simulink model "Demo3"  (Simulink 6.5)
settings: Solver=ode23t  SolverMode=SingleTasking  StartTime=0.0  StopTime=.1  RelTol=1e-3
undefined symbols (not defined in the file): powergui
libraries: powerlib x17, powerlib_extras x1
settings Model: Creator=sybille  LastModifiedBy=PC_0  ExtModeTrigMode=oneshot  ExtModeArmWhenConnect=off  ExtModeAutoUpdateStatusClock=off
settings SolverCC: MaxOrder=1
settings DataIOCC: LimitDataPoints=off  SaveOutput=off  SaveTime=off  SignalLoggingName=sigsOut
settings OptimizationCC: BlockReduction=off  BooleanDataType=off  InlineInvariantSignals=on
settings DebuggingCC: CheckExecutionContextPreStartOutputMsg=on  CheckExecutionContextRuntimeOutputMsg=on  SolverPrmCheckMsg=none  MultiTaskDSMMsg=warning  MultiTaskCondExecSysMsg=none  SigSpecEnsureSampleTimeMsg=none  UnconnectedInputMsg=none  UnconnectedOutputMsg=none  StrictBusMsg=None
settings HardwareCC: TargetUnknown=on
settings RTWCC: IncludeERTFirstTime=on

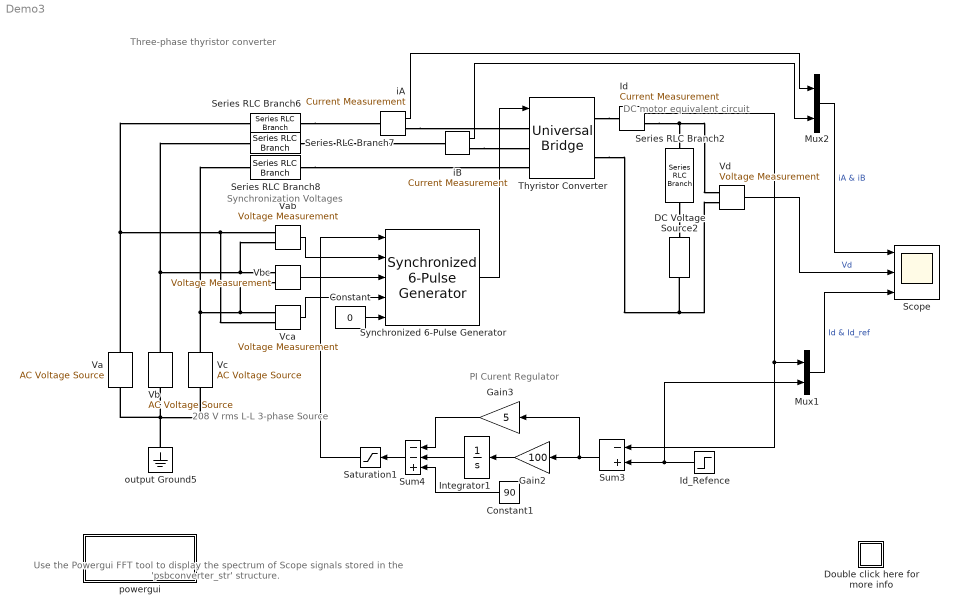
== system Demo3 ==
  note: Synchronization Voltages
  note: DC motor equivalent circuit
  note: PI Curent Regulator
  note: Three-phase thyristor converter
  note: 208 V rms L-L
      | 3-phase Source
  note: Use the Powergui FFT tool to display
      | the spectrum of Scope  signals stored in
      | the 'psbconverter_str' structure.
  Constant : Constant  Value=0  OutDataType=sfix(16)  ConRadixGroup=Use specified scaling  OutScaling=2^0  SampleTime=inf  FramePeriod=inf
  Constant1 : Constant  Orientation=left  Value=90  OutDataType=sfix(16)  ConRadixGroup=Use specified scaling  OutScaling=2^0  SampleTime=inf  FramePeriod=inf
  DC Voltage Source2 : powerlib/Electrical Sources/DC Voltage Source  Description=source block  Orientation=up  DialogController=PMDialogs.PMDefaultMaskDlg  SystemSampleTime=-1  Amplitude=120  Measurements=None
      settings: AttributesFormatString=\n
  Double click here for more info : Subsystem
      settings: OpenFcn=showdemo(bdroot(gcb))
      mask Display: disp('?')
  Gain2 : Gain  Orientation=left  Gain=100  SaturateOnIntegerOverflow=on
  Gain3 : Gain  Orientation=left  Gain=5  SaturateOnIntegerOverflow=on
  Id : powerlib/Measurements/Current Measurement  Tag=PoWeRsYsTeMmEaSuReMeNt  DialogController=PMDialogs.PMDefaultMaskDlg  SystemSampleTime=-1  PhasorSimulation=off  OutputType=Complex  PSBequivalent=0
  Id_Refence : Step  Orientation=left  Time=0.04  Before=10  After=25  SampleTime=0
  Integrator1 : Integrator  Orientation=left  InitialCondition=20  LimitOutput=on  UpperSaturationLimit=160  LowerSaturationLimit=20
  Mux1 : Mux  Inputs=2
  Mux2 : Mux  Inputs=2
  Saturation1 : Saturate  Orientation=left  UpperLimit=160  LowerLimit=20
  Scope : Scope  NumInputPorts=3
      settings: TimeRange=0.1  YMin=-50~-200~-3.20216e-017  YMax=50~400~40  SaveName=psbconverter_str  SampleInput=on  SampleTime=1/60/512
  Series RLC Branch2 : powerlib/Elements/Series RLC Branch  Orientation=down  DialogController=PMDialogs.PMDefaultMaskDlg  PhysicalDomain=powersysdomain  SubClassName=unknown  LeftPortType=p1  RightPortType=p1  LConnTagsString=__new0  RConnTagsString=__new0  BranchType=RL  Resistance=1  Inductance=20e-3  SetiL0=off  InitialCurrent=0  Capacitance=[]  Setx0=off  InitialVoltage=0  Measurements=None
  Series RLC Branch6 : powerlib/Elements/Series RLC Branch  DialogController=PMDialogs.PMDefaultMaskDlg  PhysicalDomain=powersysdomain  SubClassName=unknown  LeftPortType=p1  RightPortType=p1  LConnTagsString=__new0  RConnTagsString=__new0  BranchType=RL  Resistance=0.01  Inductance=1e-3  SetiL0=off  InitialCurrent=0  Capacitance=[]  Setx0=off  InitialVoltage=0  Measurements=None
  Series RLC Branch7 : powerlib/Elements/Series RLC Branch  DialogController=PMDialogs.PMDefaultMaskDlg  PhysicalDomain=powersysdomain  SubClassName=unknown  LeftPortType=p1  RightPortType=p1  LConnTagsString=__new0  RConnTagsString=__new0  BranchType=RL  Resistance=0.01  Inductance=1e-3  SetiL0=off  InitialCurrent=0  Capacitance=[]  Setx0=off  InitialVoltage=0  Measurements=None
  Series RLC Branch8 : powerlib/Elements/Series RLC Branch  DialogController=PMDialogs.PMDefaultMaskDlg  PhysicalDomain=powersysdomain  SubClassName=unknown  LeftPortType=p1  RightPortType=p1  LConnTagsString=__new0  RConnTagsString=__new0  BranchType=RL  Resistance=0.01  Inductance=1e-3  SetiL0=off  InitialCurrent=0  Capacitance=[]  Setx0=off  InitialVoltage=0  Measurements=None
  Sum3 : Sum  Orientation=left  Inputs=-+  SaturateOnIntegerOverflow=on  InputSameDT=on
  Sum4 : Sum  Orientation=left  Inputs=--+  SaturateOnIntegerOverflow=on  InputSameDT=on
  Synchronized 6-Pulse Generator : powerlib_extras/Control  Blocks/Synchronized 6-Pulse Generator  DialogController=PMDialogs.PMDefaultMaskDlg  SystemSampleTime=-1  freq=60  pwidth=10  Double_Pulse=on
  Thyristor Converter : powerlib/Power Electronics/Universal Bridge  DialogController=PMDialogs.PMDefaultMaskDlg  SystemSampleTime=-1  Arms=3  SnubberResistance=500  SnubberCapacitance=.1e-6  Device=Thyristors  Ron=1e-3  Lon=0  ForwardVoltages="[  0.8  0.8  ]"  ForwardVoltage=.8  GTOparameters=[ 10e-6 , 20e-6 ]  IGBTparameters=[ 1e-6 , 2e-6 ]  Measurements=None  converterType=Rectifier
  Va : powerlib/Electrical Sources/AC Voltage Source  Description=source block  Orientation=up  DialogController=PMDialogs.PMDefaultMaskDlg  SystemSampleTime=-1  Amplitude=208*sqrt(2/3)  Phase=0  Frequency=60  SampleTime=0  Measurements=None
      settings: AttributesFormatString=\n
  Vab : powerlib/Measurements/Voltage Measurement  Tag=PoWeRsYsTeMmEaSuReMeNt  DialogController=PMDialogs.PMDefaultMaskDlg  SystemSampleTime=-1  PhasorSimulation=off  OutputType=Complex  PSBequivalent=0
  Vb : powerlib/Electrical Sources/AC Voltage Source  Description=source block  Orientation=up  DialogController=PMDialogs.PMDefaultMaskDlg  SystemSampleTime=-1  Amplitude=208*sqrt(2/3)  Phase=-120  Frequency=60  SampleTime=0  Measurements=None
      settings: AttributesFormatString=\n
  Vbc : powerlib/Measurements/Voltage Measurement  Tag=PoWeRsYsTeMmEaSuReMeNt  DialogController=PMDialogs.PMDefaultMaskDlg  SystemSampleTime=-1  PhasorSimulation=off  OutputType=Complex  PSBequivalent=0
  Vc : powerlib/Electrical Sources/AC Voltage Source  Description=source block  Orientation=up  DialogController=PMDialogs.PMDefaultMaskDlg  SystemSampleTime=-1  Amplitude=208*sqrt(2/3)  Phase=120  Frequency=60  SampleTime=0  Measurements=None
      settings: AttributesFormatString=\n
  Vca : powerlib/Measurements/Voltage Measurement  Tag=PoWeRsYsTeMmEaSuReMeNt  DialogController=PMDialogs.PMDefaultMaskDlg  SystemSampleTime=-1  PhasorSimulation=off  OutputType=Complex  PSBequivalent=0
  Vd : powerlib/Measurements/Voltage Measurement  Tag=PoWeRsYsTeMmEaSuReMeNt  DialogController=PMDialogs.PMDefaultMaskDlg  SystemSampleTime=-1  PhasorSimulation=off  OutputType=Complex  PSBequivalent=0
  iA : powerlib/Measurements/Current Measurement  Tag=PoWeRsYsTeMmEaSuReMeNt  DialogController=PMDialogs.PMDefaultMaskDlg  SystemSampleTime=-1  PhasorSimulation=off  OutputType=Complex  PSBequivalent=0
  iB : powerlib/Measurements/Current Measurement  Tag=PoWeRsYsTeMmEaSuReMeNt  DialogController=PMDialogs.PMDefaultMaskDlg  SystemSampleTime=-1  PhasorSimulation=off  OutputType=Complex  PSBequivalent=0
  output Ground5 : powerlib/Elements/Ground  Orientation=down  DialogController=PMDialogs.PMDefaultMaskDlg  PhysicalDomain=powersysdomain  SubClassName=unknown  LeftPortType=p1  RightPortType=p1  LConnTagsString=a
  powergui : Subsystem  Priority=2  AncestorBlock=powerlib/powergui  InitFcn=powergui( 'InitFcn_Callback' , gcb , 0 , [ ] );  mask(PSB option menu block){SimulationMode=Continuous, SampleTime=0, echomessages=off, RestoreLinks=warning, x0status=blocks, Frange=[0:2:500], Ylog=off, Xlog=on, ShowGrid=off, save=off, variable=ZData, structure=psbconverter_str, ZoomFFT=on, StartTime=0.1-2/60, cycles=2, DisplayStyle=off, fundamental=60, FreqAxis=on, MaxFrequency=2000, frequencyindice=60, frequencyindicesteady=1, RmsSteady=1, display=off, Ts=0, frequency=60, methode=off, HookPort=off, Interpol=off}
      mask prompts: SimulationMode "Simulation mode"; SampleTime "Sample time Ts (when simulation mode is Discrete) (s)"; echomessages "Echo  Messages"; RestoreLinks "Restore disabled links"; x0status "Initial electrical states status"; Frange "Impedance tool: Frequency Range"; Ylog "Impedance tool: Log impedance"; Xlog "Impedance tool: log Frequency"; ShowGrid "Impedance tool: grid"; save "Impedance tool: Save Data To Workspace"; variable "Impedance tool: Variable Name"; structure "Structure Name (PSBFFTSCOPE)"; ZoomFFT "ZoomFFT (PSBFFTSCOPE)"; StartTime "Start Time (PSBFFTSCOPE)"; cycles "Cycles (PSBFFTSCOPE)"; DisplayStyle "Display style (PSBFFTSCOPE)"; fundamental "Fundamental (PSBFFTSCOPE)"; FreqAxis "Frequency Axis (PSBFFTSCOPE)"; MaxFrequency "Max Frequency (PSBFFTSCOPE)"; frequencyindice "Load flow frequency (Hz)"; frequencyindicesteady "Frequency indice (STEADYSTATE)"; RmsSteady "RMS display (STEADYSTATE)"; display "Display Results"; Ts "OBSOLETE 1"; frequency "Phasor frequency (Hz)"; methode "Phasor simulation"; HookPort "Hook port"; Interpol "Interpolate"
      mask init:
      | powerlibroot = which('powersysdomain');
      | PSBroot = powerlibroot(1:end-16);
      | %
      | switch SimulationMode
      | 	case 1
      | 		message=sprintf('Continuous');
      | 	case 2
      |         SampleTimeeval=evalin('base',SampleTime,'NaN');
      |         if isnan(SampleTimeeval)
      |             message=sprintf('Warning !!,\nUndefined sample time');
      |         else
      |             message=sprintf('Discrete,\nTs = %.4g s.',SampleTimeeval);
      |         end
      | 	case 3
      | 		message=sprintf('Phasors');
      | end
      | if strcmp(bdroot,'powerlib')
      |   message='powergui';
      | end
      | power_initmask();
      settings: CopyFcn=powergui( 'Copy_Callback' , gcb , 0 , [ ] );  ModelCloseFcn=powergui( 'CloseButton_Callback' , gcb , [ ] , [ ] );  PreSaveFcn=powergui( 'CloseButton_Callback' , gcb , [ ] , [ ] );  NameChangeFcn=powergui( 'NameChangeFcn_Callback' , gcb , 0 , [ ] );
      settings: DeleteFcn=|
      | powergui( 'Copy_Callback' , gcb , 1 , [ ] );
      | powergui( 'CloseButton_Callback' , gcb , [ ] , [ ] );
      settings: OpenFcn=|
      | if (power_openblockproxy ('secondary'))
      | powergui(gcb,'PM')
      | end;
      mask Help: web(psbhelp)
      mask StyleString: popup(Continuous|Discrete|Phasor),edit,checkbox,popup(yes|warning|no),popup(blocks|steady|zero),edit,checkbox,checkbox,checkbox,checkbox,edit,edit,checkbox,edit,edit,edit,edit,checkbox,edit,edit,edit,edit,checkbox,edit,edit,checkbox,checkbox,checkbox
      mask CallbackString: ||||||||||||||||||||||||||powergui('HookPort',[],[],gcb);|
      mask Display: disp(message)
  wires:
  Gain3/1 -> Sum4/1
  Constant1/1 -> Sum4/3
  Gain2/1 -> Integrator1/1
  Sum3/1 -> Gain3/1, Gain2/1
  Sum4/1 -> Saturation1/1
  Integrator1/1 -> Sum4/2
  Saturation1/1 -> Synchronized 6-Pulse Generator/1
  Id_Refence/1 -> Sum3/2, Mux1/2
  Mux2/1 -> Scope/1  "iA & iB"
  Mux1/1 -> Scope/3  "Id & Id_ref"
  Constant/1 -> Synchronized 6-Pulse Generator/5
  Id/1 -> Mux1/1, Sum3/1
  Vca/1 -> Synchronized 6-Pulse Generator/4
  Vbc/1 -> Synchronized 6-Pulse Generator/3
  Vab/1 -> Synchronized 6-Pulse Generator/2
  iA/1 -> Mux2/1
  iB/1 -> Mux2/2
  Vd/1 -> Scope/2  "Vd"
  Synchronized 6-Pulse Generator/1 -> Thyristor Converter/1
  connections:
  Thyristor Converter/RConn1 -- Id/LConn1
  output Ground5/LConn1 -- Vb/LConn1 -- Va/LConn1 -- Vc/LConn1
  Id/RConn1 -- Series RLC Branch2/LConn1 -- Vd/LConn1
  Series RLC Branch2/RConn1 -- DC Voltage Source2/RConn1
  Vb/RConn1 -- Vbc/LConn1 -- Vab/LConn2 -- Series RLC Branch7/LConn1
  Vc/RConn1 -- Vca/LConn1 -- Vbc/LConn2 -- Series RLC Branch8/LConn1
  Va/RConn1 -- Vab/LConn1 -- Vca/LConn2 -- Series RLC Branch6/LConn1
  Series RLC Branch8/RConn1 -- Thyristor Converter/LConn3
  Series RLC Branch6/RConn1 -- iA/LConn1
  iA/RConn1 -- Thyristor Converter/LConn1
  Series RLC Branch7/RConn1 -- iB/LConn1
  iB/RConn1 -- Thyristor Converter/LConn2
  Thyristor Converter/RConn2 -- DC Voltage Source2/LConn1 -- Vd/LConn2

== system Demo3/Double click here for more info ==
  note: This demonstration illustrates use of the Universal Bridge block to simulate a three-phase six-pulse
      | converter and harmonic analysis using the Powergui/FFT tool.
  note: Circuit Description
  note: A  DC motor  represented by a simplified RL-E model is fed from  an inductive three-phase source through a six-pulse
      | thyristor bridge. A pulse generator synchronized on the source voltages provides the trigger pulses for the six thyristors.
      |
      | The converter output current is controlled by a PI current regulator built with Simulink blocks.
      | A step signal is applied to the reference input to test the dynamic response of the current regulator.
      |
      | In order to allow further signal processing, signals displayed on the Scope block are sampled at 1/60/512 s (512 samples/ cycle) and stored
      | in a variable named 'psbconveter_str'  ('structure with time'  format) .
  note: H. Le-Huy (Universite Laval, Quebec)
  note: Demonstration
  note: Start simulation and observe current and voltage waveforms on the Scope block.
      |
      | When  simulation is completed, open the Powergui and select  'FFT Analysis' to display the 0 - 2000 Hz frequency spectrum of signals saved
      | in the 'psbconverter_str' structure. The FFT will be performed on  a 2-cycle window starting at t = 0.1 - 2/60 (last 2 cycles of recording).
      | Input labeled 'Ia & Ib' and signal number 1 (Ia) should be already selected. Click on Display and observe the frequency spectrum of last two cycles of Ia.
      | Harmonic currents (6n+/-1) are displayed in % of the fundamental component .
      |
      | The value of the fundamental current (magnitude = 27.48 A peak) and the Total Harmonic Distortion (THD) are also displayed.
      | Harrmonics in the 0 - 2000 Hz range contribute to 29% in THD. If you specify a 0-4000 Hz frequence range, notice that
      | contributions of harmonics above 2000 Hz are negligible in the current THD.
      |
      | Now select the input labeled Vd and display its spectrum.
      | The DC voltage contains harmonics (6n) and its DC component is 145.4 V.

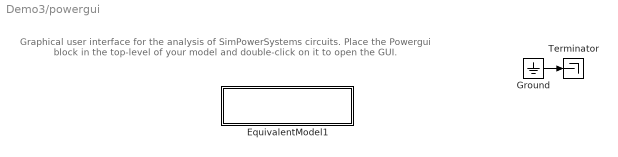
== system Demo3/powergui ==
  note: Graphical user interface for the analysis of  SimPowerSystems circuits.
      | Place the Powergui block in the top-level of your model and double-click
      | on it to open the GUI.
  EquivalentModel1 : Subsystem
      mask init:
      | SPS = get_param(gcbh,'UserData');
      | if isempty(SPS)
      |     A=0;
      |     B=0;
      |     C=0;
      |     D=0;
      |     x0=0;
      |     SwitchResistance=1;
      |     SwitchType=1;
      |     SwitchGateInitialValue=1;
      |     OutputsToResetToZero=1;
      | else
      | 	A=SPS.A;
      |     B=SPS.B;
      |     C=SPS.C;
      |     D=SPS.D;
      |     x0=SPS.x0;
      |     SwitchResistance=SPS.SwitchResistance;
      |     SwitchType=SPS.SwitchType;
      |     SwitchGateInitialValue=SPS.SwitchGateInitialValue;
      |     OutputsToResetToZero=SPS.YSwitchCurrent;
      | end
      mask Display:
      | color('blue')
      | disp('EQUIVALENT CIRCUIT')
  Ground : Ground
  Terminator : Terminator
  wires:
  Ground/1 -> Terminator/1

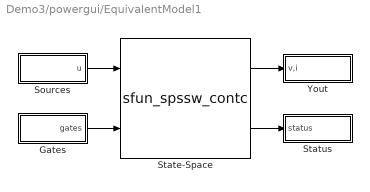
== system Demo3/powergui/EquivalentModel1 ==
  Gates : Subsystem
  Sources : Subsystem
  State-Space : S-Function  FunctionName=sfun_spssw_contc  Parameters=A, B, C, D, x0, SwitchResistance ,SwitchType, SwitchGateInitialValue, OutputsToResetToZero
  Status : Subsystem
  Yout : Subsystem
  wires:
  Gates/1(gates) -> State-Space/2
  Sources/1(u) -> State-Space/1
  State-Space/2 -> Status/1(status)
  State-Space/1 -> Yout/1(v,i)

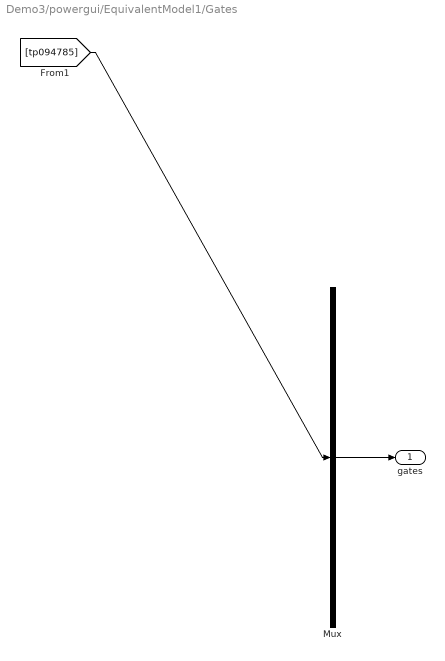
== system Demo3/powergui/EquivalentModel1/Gates ==
  Mux : Mux  Inputs=1
  gates : Outport
  wires:
  Mux/1 -> gates/1
  [tp094785] -> Mux/1

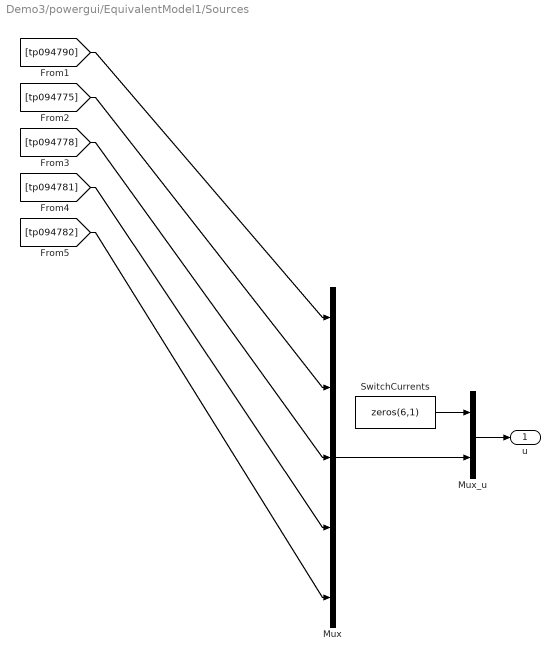
== system Demo3/powergui/EquivalentModel1/Sources ==
  Mux : Mux  Inputs=[1 1 1 1 6]
  Mux_u : Mux  Inputs=[6 10]
  SwitchCurrents : Constant  Value=zeros(6,1)  OutDataType=sfix(16)  ConRadixGroup=Use specified scaling  OutScaling=2^0  SampleTime=inf  FramePeriod=inf
  u : Outport
  wires:
  Mux/1 -> Mux_u/2
  SwitchCurrents/1 -> Mux_u/1
  Mux_u/1 -> u/1
  [tp094790] -> Mux/1
  [tp094775] -> Mux/2
  [tp094778] -> Mux/3
  [tp094781] -> Mux/4
  [tp094782] -> Mux/5

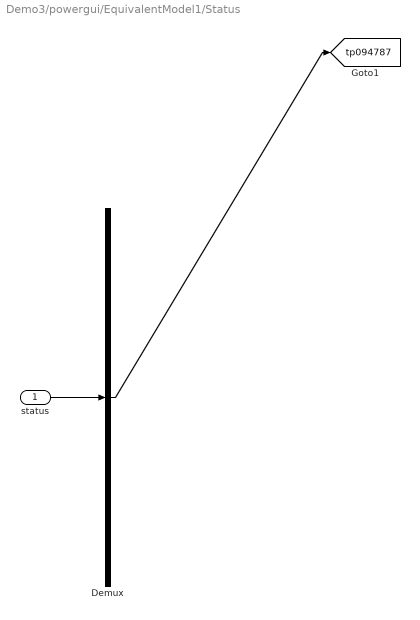
== system Demo3/powergui/EquivalentModel1/Status ==
  status : Inport
  Demux : Demux  Outputs=1
  tag scope: tp094787=global
  wires:
  status/1 -> Demux/1
  Demux/1 -> [tp094787]

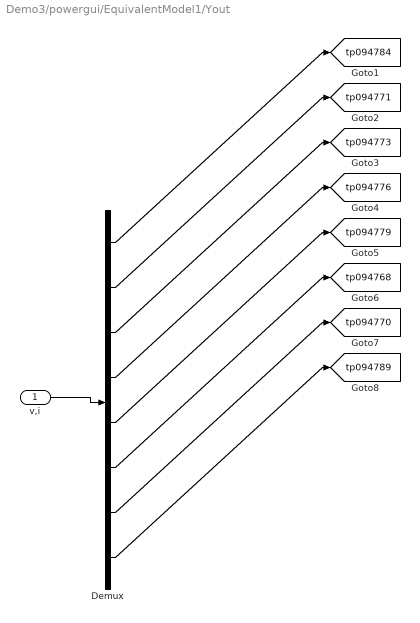
== system Demo3/powergui/EquivalentModel1/Yout ==
  v,i : Inport
  Demux : Demux  Outputs=[6 1 1 1 1 1 1 1]
  tag scope: tp094768=global, tp094770=global, tp094771=global, tp094773=global, tp094776=global, tp094779=global, tp094784=global, tp094789=global
  wires:
  v,i/1 -> Demux/1
  Demux/1 -> [tp094784]
  Demux/2 -> [tp094771]
  Demux/3 -> [tp094773]
  Demux/4 -> [tp094776]
  Demux/5 -> [tp094779]
  Demux/6 -> [tp094768]
  Demux/7 -> [tp094770]
  Demux/8 -> [tp094789]
